simulink model "untitled"  (R2018b)
settings: Solver=VariableStepAuto  StartTime=0.0  StopTime=10.0  RelTol=1e-3
values from neighbouring files (symbols this model uses):
  BOT1_pos = zeros(3,length(t))    [Tetrahedron_Based_Relative_Localization.m]
  bot1_transmitted = zeros(3,length(t))    [Transmission_Channal.m]
  bot2_transmitted = zeros(3,length(t))    [Transmission_Channal.m]
  bot3_transmitted = zeros(3,length(t))    [Transmission_Channal.m]
  bot4_transmitted = zeros(3,length(t))    [Transmission_Channal.m]
undefined symbols (not defined in the file or in its folder): smiData, X, Y, Z
libraries: simulink x15, nesl_utility x6, sm_lib x5
settings Model: Creator=Yogesh  LastModifiedBy=Yogesh

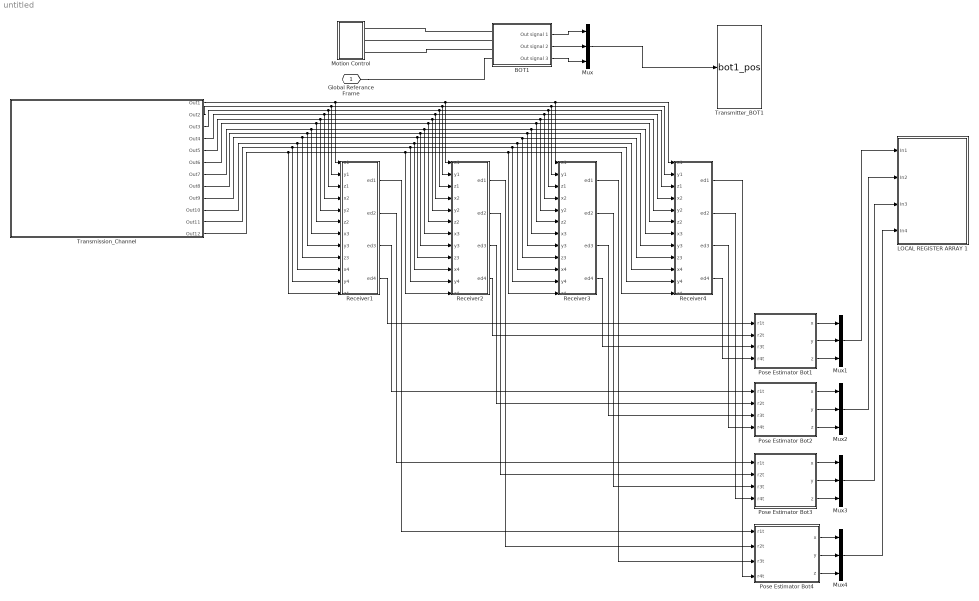
== system untitled ==
  BOT1 : Subsystem
  LOCAL REGISTER ARRAY 1 : Subsystem
  Motion Control : Subsystem
  Mux{,1..4} (5 alike) : Mux  Inputs=3
  Pose Estimator Bot1 : MATLAB Function  TreatAsAtomicUnit=on
  Pose Estimator Bot2 : MATLAB Function  TreatAsAtomicUnit=on
  Pose Estimator Bot3 : MATLAB Function  TreatAsAtomicUnit=on
  Pose Estimator Bot4 : MATLAB Function  TreatAsAtomicUnit=on
  Receiver1 : MATLAB Function  TreatAsAtomicUnit=on
  Receiver2 : MATLAB Function  TreatAsAtomicUnit=on
  Receiver3 : MATLAB Function  TreatAsAtomicUnit=on
  Receiver4 : MATLAB Function  TreatAsAtomicUnit=on
  Transmission_Channel : Subsystem
  Transmitter_BOT1 : ToWorkspace  VariableName=bot1_pos  SampleTime=-1
  Global Referance Frame : PMIOPort  Side=Left
  wires:
  Pose Estimator Bot3/1(x) -> Mux3/1
  Pose Estimator Bot2/1(x) -> Mux2/1
  Pose Estimator Bot3/2(y) -> Mux3/2
  Mux/1 -> Transmitter_BOT1/1
  Mux4/1 -> LOCAL REGISTER ARRAY 1/4(In4)
  Mux2/1 -> LOCAL REGISTER ARRAY 1/2(In2)
  Mux3/1 -> LOCAL REGISTER ARRAY 1/3(In3)
  Mux1/1 -> LOCAL REGISTER ARRAY 1/1(In1)
  Pose Estimator Bot4/3(z) -> Mux4/3
  Pose Estimator Bot2/3(z) -> Mux2/3
  Pose Estimator Bot1/1(x) -> Mux1/1
  Pose Estimator Bot3/3(z) -> Mux3/3
  Pose Estimator Bot4/2(y) -> Mux4/2
  Pose Estimator Bot1/2(y) -> Mux1/2
  Pose Estimator Bot4/1(x) -> Mux4/1
  Pose Estimator Bot2/2(y) -> Mux2/2
  Pose Estimator Bot1/3(z) -> Mux1/3
  BOT1/1(Out signal 1) -> Mux/1
  BOT1/2(Out signal 2) -> Mux/2
  BOT1/3(Out signal 3) -> Mux/3
  Transmission_Channel/6(Out6) -> Receiver1/6(z2), Receiver2/6(z2), Receiver3/6(z2), Receiver4/6(z2)
  Transmission_Channel/4(Out4) -> Receiver1/4(x2), Receiver2/4(x2), Receiver4/4(x2), Receiver3/4(x2)
  Transmission_Channel/2(Out2) -> Receiver1/2(y1), Receiver2/2(y1), Receiver4/2(y1), Receiver3/2(y1)
  Transmission_Channel/11(Out11) -> Receiver1/11(y4), Receiver2/11(y4), Receiver4/11(y4), Receiver3/11(y4)
  Transmission_Channel/3(Out3) -> Receiver1/3(z1), Receiver2/3(z1), Receiver4/3(z1), Receiver3/3(z1)
  Transmission_Channel/1(Out1) -> Receiver1/1(x1), Receiver2/1(x1), Receiver4/1(x1), Receiver3/1(x1)
  Transmission_Channel/9(Out9) -> Receiver1/9(z3), Receiver2/9(z3), Receiver4/9(z3), Receiver3/9(z3)
  Transmission_Channel/5(Out5) -> Receiver1/5(y2), Receiver2/5(y2), Receiver4/5(y2), Receiver3/5(y2)
  Transmission_Channel/12(Out12) -> Receiver1/12(z4), Receiver2/12(z4), Receiver4/12(z4), Receiver3/12(z4)
  Transmission_Channel/10(Out10) -> Receiver1/10(x4), Receiver2/10(x4), Receiver4/10(x4), Receiver3/10(x4)
  Transmission_Channel/8(Out8) -> Receiver1/8(y3), Receiver2/8(y3), Receiver4/8(y3), Receiver3/8(y3)
  Transmission_Channel/7(Out7) -> Receiver1/7(x3), Receiver2/7(x3), Receiver4/7(x3), Receiver3/7(x3)
  Receiver1/1(ed1) -> Pose Estimator Bot4/1(r1t)
  Receiver1/2(ed2) -> Pose Estimator Bot3/1(r1t)
  Receiver1/3(ed3) -> Pose Estimator Bot2/1(r1t)
  Receiver1/4(ed4) -> Pose Estimator Bot1/1(r1t)
  Receiver2/1(ed1) -> Pose Estimator Bot4/2(r2t)
  Receiver2/2(ed2) -> Pose Estimator Bot3/2(r2t)
  Receiver2/3(ed3) -> Pose Estimator Bot2/2(r2t)
  Receiver2/4(ed4) -> Pose Estimator Bot1/2(r2t)
  Receiver3/1(ed1) -> Pose Estimator Bot4/3(r3t)
  Receiver3/2(ed2) -> Pose Estimator Bot3/3(r3t)
  Receiver3/3(ed3) -> Pose Estimator Bot2/3(r3t)
  Receiver3/4(ed4) -> Pose Estimator Bot1/3(r3t)
  Receiver4/1(ed1) -> Pose Estimator Bot4/4(r4t)
  Receiver4/2(ed2) -> Pose Estimator Bot3/4(r4t)
  Receiver4/3(ed3) -> Pose Estimator Bot2/4(r4t)
  Receiver4/4(ed4) -> Pose Estimator Bot1/4(r4t)
  connections:
  BOT1/LConn1 -- Motion Control/RConn1
  BOT1/LConn2 -- Motion Control/RConn2
  BOT1/LConn3 -- Motion Control/RConn3
  Global Referance Frame/RConn1 -- BOT1/LConn4

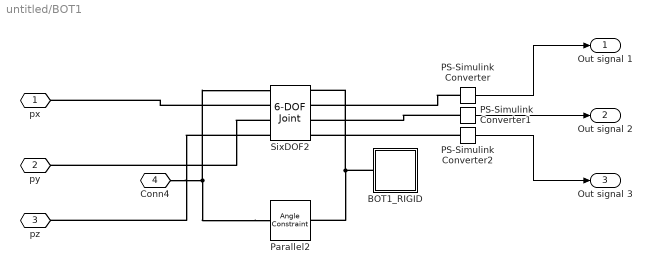
== system untitled/BOT1 ==
  BOT1_RIGID : Subsystem
  PS-Simulink Converter : nesl_utility/PS-Simulink Converter  PhysicalDomain=network_engine_domain  SubClassName=ps_output  LeftPortType=input  RightPortType=output  PseudoPeriodic=off  Frequencies=[]  Unit=m  AffineConversion=off
  PS-Simulink Converter1 : nesl_utility/PS-Simulink Converter  PhysicalDomain=network_engine_domain  SubClassName=ps_output  LeftPortType=input  RightPortType=output  PseudoPeriodic=off  Frequencies=[]  Unit=m  AffineConversion=off
  PS-Simulink Converter2 : nesl_utility/PS-Simulink Converter  PhysicalDomain=network_engine_domain  SubClassName=ps_output  LeftPortType=input  RightPortType=output  PseudoPeriodic=off  Frequencies=[]  Unit=m  AffineConversion=off
  Parallel2 : sm_lib/Constraints/Angle Constraint  ConstraintType=Parallel  Angle=45  AngleUnits=deg  SenseSignedTorqueMagnitude=off  SenseTorque=off  SenseForce=off  WrenchDir=FollowerOnBase  WrenchFrame=BaseFrame
      settings: SourceProductName=Simscape Multibody  SourceProductBaseCode=MS
  SixDOF2 : sm_lib/Joints/6-DOF Joint  SenseConstraintForce=off  SenseConstraintForceX=off  SenseConstraintForceY=off  SenseConstraintForceZ=off  SenseConstraintTorque=off  SenseConstraintTorqueX=off  SenseConstraintTorqueY=off  SenseConstraintTorqueZ=off  SenseTotalForce=off  SenseTotalForceX=off  SenseTotalForceY=off  SenseTotalForceZ=off  SenseTotalTorque=off  SenseTotalTorqueX=off  SenseTotalTorqueY=off  SenseTotalTorqueZ=off  CompositeWrenchDir=FollowerOnBase  CompositeWrenchFrame=BaseFrame  PxEquilibriumPosition=0  PxEquilibriumPositionUnits=m  PxSpringStiffness=0  PxSpringStiffnessUnits=N/m  PxDampingCoefficient=0  PxDampingCoefficientUnits=N/(m/s)  PxTorqueActuationMode=ComputedTorque  PxMotionActuationMode=InputMotion  PxSensePosition=on  PxSenseVelocity=off  PxSenseAcceleration=off  PxSenseTorqueForce=off  PxPositionTargetSpecify=on  PxPositionTargetPriority=Low  PxPositionTargetValue=smiData.SixDofJoint(3).Px.Pos  PxPositionTargetValueUnits=in  PxVelocityTargetSpecify=off  PxVelocityTargetPriority=High  PxVelocityTargetValue=0  PxVelocityTargetValueUnits=m/s  PyEquilibriumPosition=0  PyEquilibriumPositionUnits=m  PySpringStiffness=0  PySpringStiffnessUnits=N/m  PyDampingCoefficient=0  PyDampingCoefficientUnits=N/(m/s)  PyTorqueActuationMode=ComputedTorque  PyMotionActuationMode=InputMotion  PySensePosition=on  PySenseVelocity=off  PySenseAcceleration=off  PySenseTorqueForce=off  PyPositionTargetSpecify=on  PyPositionTargetPriority=Low  PyPositionTargetValue=smiData.SixDofJoint(3).Py.Pos  PyPositionTargetValueUnits=in  PyVelocityTargetSpecify=off  PyVelocityTargetPriority=High  PyVelocityTargetValue=0  PyVelocityTargetValueUnits=m/s  PzEquilibriumPosition=0  PzEquilibriumPositionUnits=m  PzSpringStiffness=0  PzSpringStiffnessUnits=N/m  PzDampingCoefficient=0  PzDampingCoefficientUnits=N/(m/s)  PzTorqueActuationMode=ComputedTorque  PzMotionActuationMode=InputMotion  PzSensePosition=on  PzSenseVelocity=off  PzSenseAcceleration=off  PzSenseTorqueForce=off  PzPositionTargetSpecify=on  PzPositionTargetPriority=Low  PzPositionTargetValue=smiData.SixDofJoint(3).Pz.Pos  PzPositionTargetValueUnits=in  PzVelocityTargetSpecify=off  PzVelocityTargetPriority=High  PzVelocityTargetValue=0  PzVelocityTargetValueUnits=m/s  SphDefPosRotationMethod=None  SphDefPosRotationAngleUnits=deg  SphDefPosRotationStandardAxis=+Z  SphDefPosRotationAngle=0.0  SphDefPosRotationArbitraryAxis=[0 0 1]  SphDefPosFollAlignAxisA=+X  SphDefPosBaseAlignAxisA=+Y  SphDefPosFollAlignAxisB=+Y  SphDefPosBaseAlignAxisB=+Z  SphDefPosRotationSequenceAxes=FollowerAxes  SphDefPosRotationSequence=XYX  SphDefPosRotationSequenceAngles=[0 0 0]  SphDefPosRotationSequenceAnglesUnits=deg  SphDefPosRotationMatrix=[1 0 0; 0 1 0; 0 0 1]  SphEqPosRotationMethod=None  SphEqPosRotationAngleUnits=deg  SphEqPosRotationStandardAxis=+Z  SphEqPosRotationAngle=0.0  SphEqPosRotationArbitraryAxis=[0 0 1]  SphEqPosFollAlignAxisA=+X  SphEqPosBaseAlignAxisA=+Y  SphEqPosFollAlignAxisB=+Y  SphEqPosBaseAlignAxisB=+Z  SphEqPosRotationSequenceAxes=FollowerAxes  SphEqPosRotationSequence=XYX  SphEqPosRotationSequenceAngles=[0 0 0]  SphEqPosRotationSequenceAnglesUnits=deg  SphEqPosRotationMatrix=[1 0 0; 0 1 0; 0 0 1]  SphSpringStiffness=0  SphSpringStiffnessUnits=N*m/rad  SphDampingCoefficient=0  SphDampingCoefficientUnits=N*m/(rad/s)  SphActuateTorqueX=off  SphActuateTorqueY=off  SphActuateTorqueZ=off  SphActuateTorque=off  SphTorqueActuationMode=NoTorque  SphMotionActuationMode=ComputedMotion  SphActuationFrame=BaseFrame  SphSensePosition=off  SphSenseVelocityX=off  SphSenseVelocityY=off  SphSenseVelocityZ=off  SphSenseVelocity=off  SphSenseAccelerationX=off  SphSenseAccelerationY=off  SphSenseAccelerationZ=off  SphSenseAcceleration=off  SphSenseTorqueX=off  SphSenseTorqueY=off  SphSenseTorqueZ=off  SphSenseTorqueForce=off  SphSensingFrame=FollowerFrame  SphPositionTargetRotationMethod=ArbitraryAxis  SphPositionTargetRotationAngleUnits=deg  SphPositionTargetRotationStandardAxis=+Z  SphPositionTargetRotationAngle=smiData.SixDofJoint(3).S.Pos.Angle  SphPositionTargetRotationArbitraryAxis=smiData.SixDofJoint(3).S.Pos.Axis  SphPositionTargetFollAlignAxisA=+X  SphPositionTargetBaseAlignAxisA=+Y  SphPositionTargetFollAlignAxisB=+Y  SphPositionTargetBaseAlignAxisB=+Z  SphPositionTargetRotationSequenceAxes=FollowerAxes  SphPositionTargetRotationSequence=XYX  SphPositionTargetRotationSequenceAngles=[0 0 0]  SphPositionTargetRotationSequenceAnglesUnits=deg  SphPositionTargetRotationMatrix=[1 0 0; 0 1 0; 0 0 1]  SphPositionTargetSpecify=on  SphPositionTargetPriority=Low  SphVelocityTargetValue=[0 0 0]  SphVelocityTargetValueUnits=deg/s  SphVelocityTargetSpecify=off  SphVelocityTargetPriority=High  SphVelocityTargetInFollowerFrame=on
  px : PMIOPort  Side=Left
  py : PMIOPort  Port=2  Side=Left
  pz : PMIOPort  Port=3  Side=Left
  Conn4 : PMIOPort  Port=4  Side=Left
  Out signal 1 : Outport
  Out signal 2 : Outport  Port=2
  Out signal 3 : Outport  Port=3
  wires:
  PS-Simulink Converter/1 -> Out signal 1/1
  PS-Simulink Converter1/1 -> Out signal 2/1
  PS-Simulink Converter2/1 -> Out signal 3/1
  connections:
  SixDOF2/RConn1 -- BOT1_RIGID/LConn1 -- Parallel2/RConn1
  SixDOF2/LConn2 -- px/RConn1
  PS-Simulink Converter1/LConn1 -- SixDOF2/RConn3
  Parallel2/LConn1 -- Conn4/RConn1 -- SixDOF2/LConn1
  PS-Simulink Converter/LConn1 -- SixDOF2/RConn2
  PS-Simulink Converter2/LConn1 -- SixDOF2/RConn4
  SixDOF2/LConn3 -- py/RConn1
  SixDOF2/LConn4 -- pz/RConn1

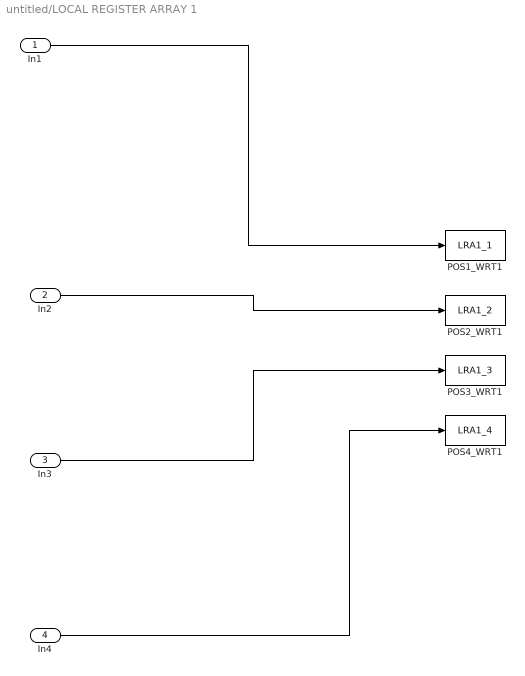
== system untitled/LOCAL REGISTER ARRAY 1 ==
  In1 : Inport
  In2 : Inport  Port=2
  In3 : Inport  Port=3
  In4 : Inport  Port=4
  POS1_WRT1 : ToWorkspace  VariableName=LRA1_1  SampleTime=-1
  POS2_WRT1 : ToWorkspace  VariableName=LRA1_2  SampleTime=-1
  POS3_WRT1 : ToWorkspace  VariableName=LRA1_3  SampleTime=-1
  POS4_WRT1 : ToWorkspace  VariableName=LRA1_4  SampleTime=-1
  wires:
  In2/1 -> POS2_WRT1/1
  In3/1 -> POS3_WRT1/1
  In1/1 -> POS1_WRT1/1
  In4/1 -> POS4_WRT1/1

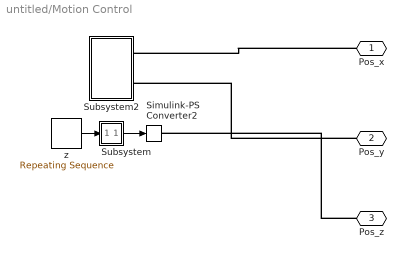
== system untitled/Motion Control ==
  Simulink-PS Converter2 : nesl_utility/Simulink-PS Converter  PhysicalDomain=network_engine_domain  SubClassName=ps_input  LeftPortType=input  RightPortType=output  PseudoPeriodic=off  Frequencies=[]  NoiseDistribution=none  NoiseParameters=[]  Unit=m  AffineConversion=off  FilteringAndDerivatives=filter  SimscapeFilterOrder=2  InputFilterTimeConstant=0.001  UdotUserProvided=0
  Subsystem : Subsystem
  Subsystem2 : Subsystem
  z : simulink/Sources/Repeating Sequence  rep_seq_t=t  rep_seq_y=BOT1_pos(3,:)
  Pos_x : PMIOPort  Side=Right
  Pos_y : PMIOPort  Port=2  Side=Right
  Pos_z : PMIOPort  Port=3  Side=Right
  wires:
  Subsystem/1(2) -> Simulink-PS Converter2/1
  z/1 -> Subsystem/1(1)
  connections:
  Pos_z/RConn1 -- Simulink-PS Converter2/RConn1
  Pos_y/RConn1 -- Subsystem2/RConn2
  Pos_x/RConn1 -- Subsystem2/RConn1

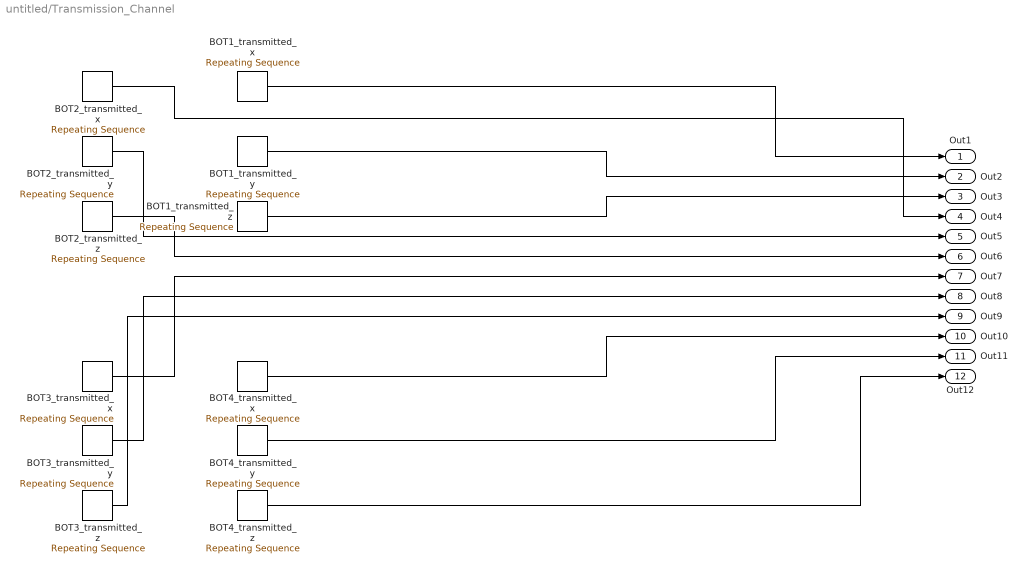
== system untitled/Transmission_Channel ==
  BOT1_transmitted_x : simulink/Sources/Repeating Sequence  rep_seq_t=t  rep_seq_y=bot1_transmitted(1,:)
  BOT1_transmitted_y : simulink/Sources/Repeating Sequence  rep_seq_t=t  rep_seq_y=bot1_transmitted(2,:)
  BOT1_transmitted_z : simulink/Sources/Repeating Sequence  rep_seq_t=t  rep_seq_y=bot1_transmitted(3,:)
  BOT2_transmitted_x : simulink/Sources/Repeating Sequence  rep_seq_t=t  rep_seq_y=bot2_transmitted(1,:)
  BOT2_transmitted_y : simulink/Sources/Repeating Sequence  rep_seq_t=t  rep_seq_y=bot2_transmitted(2,:)
  BOT2_transmitted_z : simulink/Sources/Repeating Sequence  rep_seq_t=t  rep_seq_y=bot2_transmitted(3,:)
  BOT3_transmitted_x : simulink/Sources/Repeating Sequence  rep_seq_t=t  rep_seq_y=bot3_transmitted(1,:)
  BOT3_transmitted_y : simulink/Sources/Repeating Sequence  rep_seq_t=t  rep_seq_y=bot3_transmitted(2,:)
  BOT3_transmitted_z : simulink/Sources/Repeating Sequence  rep_seq_t=t  rep_seq_y=bot3_transmitted(3,:)
  BOT4_transmitted_x : simulink/Sources/Repeating Sequence  rep_seq_t=t  rep_seq_y=bot4_transmitted(1,:)
  BOT4_transmitted_y : simulink/Sources/Repeating Sequence  rep_seq_t=t  rep_seq_y=bot4_transmitted(2,:)
  BOT4_transmitted_z : simulink/Sources/Repeating Sequence  rep_seq_t=t  rep_seq_y=bot4_transmitted(3,:)
  Out1 : Outport
  Out2 : Outport  Port=2
  Out3 : Outport  Port=3
  Out4 : Outport  Port=4
  Out5 : Outport  Port=5
  Out6 : Outport  Port=6
  Out7 : Outport  Port=7
  Out8 : Outport  Port=8
  Out9 : Outport  Port=9
  Out10 : Outport  Port=10
  Out11 : Outport  Port=11
  Out12 : Outport  Port=12
  wires:
  BOT1_transmitted_x/1 -> Out1/1
  BOT4_transmitted_z/1 -> Out12/1
  BOT1_transmitted_z/1 -> Out3/1
  BOT3_transmitted_x/1 -> Out7/1
  BOT3_transmitted_z/1 -> Out9/1
  BOT2_transmitted_z/1 -> Out6/1
  BOT2_transmitted_y/1 -> Out5/1
  BOT3_transmitted_y/1 -> Out8/1
  BOT1_transmitted_y/1 -> Out2/1
  BOT2_transmitted_x/1 -> Out4/1
  BOT4_transmitted_x/1 -> Out10/1
  BOT4_transmitted_y/1 -> Out11/1

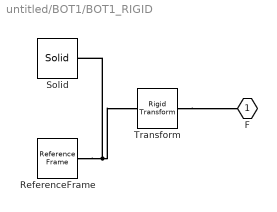
== system untitled/BOT1/BOT1_RIGID ==
  ReferenceFrame : sm_lib/Frames and Transforms/Reference Frame
  Solid : sm_lib/Body Elements/Solid  InertiaType=Custom  Mass=smiData.Solid(3).mass  MassUnits=kg  CenterOfMass=smiData.Solid(3).CoM  CenterOfMassUnits=mm  MomentsOfInertia=smiData.Solid(3).MoI  MomentsOfInertiaUnits=kg*mm^2  ProductsOfInertia=smiData.Solid(3).PoI  ProductsOfInertiaUnits=kg*mm^2  BasedOnType=Density  Density=1000  DensityUnits=kg/m^3  DoExposeReferenceFrame=on  SerializedFrames=<Frames/>  GraphicType=FromGeometry  MarkerShape=Sphere  MarkerSize=10  GraphicVisPropType=AdvancedVisualProperties  GraphicDiffuseColor=[1.0 0.2 0.2]  GraphicSpecularColor=[0.5 0.5 0.5 1.0]  GraphicAmbientColor=[0.15 0.15 0.15 1.0]  GraphicEmissiveColor=[0.0 0.0 0.0 1.0]  GraphicShininess=75  GraphicOpacity=smiData.Solid(3).opacity  GeometryShape=FromFile  RectangleSize=[1 1]  RectangleSizeUnits=m  BrickDimensions=[1 1 1]  BrickDimensionUnits=m  CylinderRadius=1  CylinderRadiusUnits=m  CylinderLength=1  CylinderLengthUnits=m  SphereRadius=1  SphereRadiusUnits=m  EllipsoidRadii=[1 1 1]  EllipsoidRadiiUnits=m  ExtrusionCrossSection=[1 1; -1 1; -1 -1; 1 -1]  ExtrusionCrossSectionUnits=m  ExtrusionLength=1  ExtrusionLengthUnits=m  PolygonNumSides=3  PolygonOuterRadius=1  PolygonOuterRadiusUnits=m  ExtGeomFileType=STEP  ExtGeomFileName=BOT3_Default_sldprt.STEP  ExtGeomFileUnits=m  RevolutionCrossSection=[1 1; 1 -1; 2 -1; 2 1]  RevolutionCrossSectionUnits=m  RevolutionExtent=Full  RevolutionAngle=180  RevolutionAngleUnits=deg
  Transform : sm_lib/Frames and Transforms/Rigid Transform  TranslationMethod=Cartesian  TranslationStandardOffset=0  TranslationLengthUnit=m  TranslationStandardAxis=+Z  TranslationCartesianOffset=smiData.RigidTransform(6).translation  TranslationROffset=0  TranslationROffsetUnits=m  TranslationZOffset=0  TranslationZOffsetUnits=m  TranslationThetaOffset=0  TranslationThetaOffsetUnits=deg  RotationMethod=ArbitraryAxis  RotationAngleUnits=rad  RotationStandardAxis=+Z  RotationAngle=smiData.RigidTransform(6).angle  RotationArbitraryAxis=smiData.RigidTransform(6).axis  FollAlignAxisA=+X  BaseAlignAxisA=+Y  FollAlignAxisB=+Y  BaseAlignAxisB=+Z  RotationSequenceAxes=FollowerAxes  RotationSequence=XYX  RotationSequenceAngles=[0 0 0]  RotationSequenceAnglesUnits=deg  RotationMatrix=[1 0 0; 0 1 0; 0 0 1]
  F : PMIOPort  Side=Left
  connections:
  Solid/RConn1 -- ReferenceFrame/RConn1 -- Transform/LConn1
  Transform/RConn1 -- F/RConn1

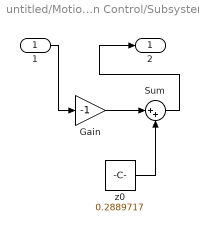
== system untitled/Motion Control/Subsystem ==
  1 : Inport
  Gain : Gain  Gain=-1
  Sum : Sum  Inputs=|++
  z0 : Constant  Value=0.2889717
  2 : Outport
  wires:
  z0/1 -> Sum/2
  Gain/1 -> Sum/1
  Sum/1 -> 2/1
  1/1 -> Gain/1

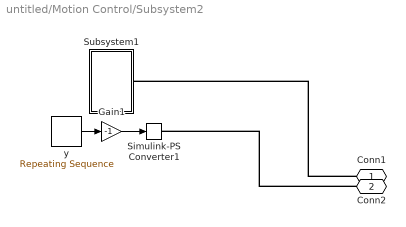
== system untitled/Motion Control/Subsystem2 ==
  Gain1 : Gain  Gain=-1
  Simulink-PS Converter1 : nesl_utility/Simulink-PS Converter  PhysicalDomain=network_engine_domain  SubClassName=ps_input  LeftPortType=input  RightPortType=output  PseudoPeriodic=off  Frequencies=[]  NoiseDistribution=none  NoiseParameters=[]  Unit=m  AffineConversion=off  FilteringAndDerivatives=filter  SimscapeFilterOrder=2  InputFilterTimeConstant=0.001  UdotUserProvided=0
  Subsystem1 : Subsystem
  y : simulink/Sources/Repeating Sequence  rep_seq_t=t  rep_seq_y=BOT1_pos(2,:)
  Conn1 : PMIOPort  Side=Right
  Conn2 : PMIOPort  Port=2  Side=Right
  wires:
  y/1 -> Gain1/1
  Gain1/1 -> Simulink-PS Converter1/1
  connections:
  Conn2/RConn1 -- Simulink-PS Converter1/RConn1
  Conn1/RConn1 -- Subsystem1/RConn1

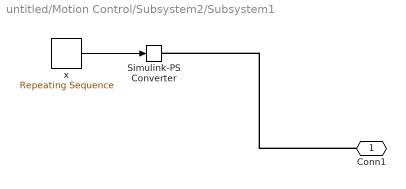
== system untitled/Motion Control/Subsystem2/Subsystem1 ==
  Simulink-PS Converter : nesl_utility/Simulink-PS Converter  PhysicalDomain=network_engine_domain  SubClassName=ps_input  LeftPortType=input  RightPortType=output  PseudoPeriodic=off  Frequencies=[]  NoiseDistribution=none  NoiseParameters=[]  Unit=m  AffineConversion=off  FilteringAndDerivatives=filter  SimscapeFilterOrder=2  InputFilterTimeConstant=0.001  UdotUserProvided=0
  x : simulink/Sources/Repeating Sequence  rep_seq_t=t  rep_seq_y=BOT1_pos(1,:)
  Conn1 : PMIOPort  Side=Right
  wires:
  x/1 -> Simulink-PS Converter/1
  connections:
  Conn1/RConn1 -- Simulink-PS Converter/RConn1

== matlab function untitled/Receiver2 ==
  data: x1 input; ed1 output; y1 input; z1 input; x2 input; y2 input; z2 input; x3 input; y3 input; z3 input; x4 input; y4 input; z4 input; ed2 output; ed3 output; ed4 output
function [ed1,ed2,ed3,ed4] = fcn(x1,y1,z1,x2,y2,z2,x3,y3,z3,x4,y4,z4)
ed1 = ((x1-x1)^2+(y1-0.57735-y1)^2+(z1+0.204124-z1)^2)^0.5;
ed2 = ((x2-x1)^2+(y2-0.57735-y1)^2+(z2+0.204124-z1)^2)^0.5;
ed3 = ((x3-x1)^2+(y3-0.57735-y1)^2+(z3+0.204124-z1)^2)^0.5;
ed4 = ((x4-x1)^2+(y4-0.57735-y1)^2+(z4+0.204124-z1)^2)^0.5;

== matlab function untitled/Receiver3 ==
  data: x1 input; ed1 output; y1 input; z1 input; x2 input; y2 input; z2 input; x3 input; y3 input; z3 input; x4 input; y4 input; z4 input; ed2 output; ed3 output; ed4 output
function [ed1,ed2,ed3,ed4] = fcn(x1,y1,z1,x2,y2,z2,x3,y3,z3,x4,y4,z4)
ed1 = ((x1-x1)^2+(y1-0.57735-y1)^2+(z1+0.204124-z1)^2)^0.5;
ed2 = ((x2-x1)^2+(y2-0.57735-y1)^2+(z2+0.204124-z1)^2)^0.5;
ed3 = ((x3-x1)^2+(y3-0.57735-y1)^2+(z3+0.204124-z1)^2)^0.5;
ed4 = ((x4-x1)^2+(y4-0.57735-y1)^2+(z4+0.204124-z1)^2)^0.5;

== matlab function untitled/Receiver4 ==
  data: x1 input; ed1 output; y1 input; z1 input; x2 input; y2 input; z2 input; x3 input; y3 input; z3 input; x4 input; y4 input; z4 input; ed2 output; ed3 output; ed4 output
function [ed1,ed2,ed3,ed4] = fcn(x1,y1,z1,x2,y2,z2,x3,y3,z3,x4,y4,z4)
ed1 = ((x1-x1)^2+(y1-0.57735-y1)^2+(z1+0.204124-z1)^2)^0.5;
ed2 = ((x2-x1)^2+(y2-0.57735-y1)^2+(z2+0.204124-z1)^2)^0.5;
ed3 = ((x3-x1)^2+(y3-0.57735-y1)^2+(z3+0.204124-z1)^2)^0.5;
ed4 = ((x4-x1)^2+(y4-0.57735-y1)^2+(z4+0.204124-z1)^2)^0.5;

== matlab function untitled/Pose Estimator Bot1 ==
  data: x output; r1t input; y output; r2t input; r3t input; r4t input; z output
function [x,y,z] = fcn(r1t,r2t,r3t,r4t)
M = [0 -3.8462 0;4.4412 2.2206 0;-1.5702 -3.3140 -4.7104];
R = [r2t^2-r1t^2;r3t^2-r2t^2;r4t^2-r3t^2];
P = M*R;
x = P(1);
y = P(2);
z = P(3);

== matlab function untitled/Pose Estimator Bot2 ==
  data: x output; r1t input; y output; r2t input; r3t input; r4t input; z output
function [x,y,z] = fcn(r1t,r2t,r3t,r4t)
M = [0 -3.8462 0;4.4412 2.2206 0;-1.5702 -3.3140 -4.7104];
R = [r2t^2-r1t^2;r3t^2-r2t^2;r4t^2-r3t^2];
P = M*R;
x = P(1);
y = P(2);
z = P(3);

== matlab function untitled/Pose Estimator Bot3 ==
  data: x output; r1t input; y output; r2t input; r3t input; r4t input; z output
function [x,y,z] = fcn(r1t,r2t,r3t,r4t)
M = [0 -3.8462 0;4.4412 2.2206 0;-1.5702 -3.3140 -4.7104];
R = [r2t^2-r1t^2;r3t^2-r2t^2;r4t^2-r3t^2];
P = M*R;
x = P(1);
y = P(2);
z = P(3);

== matlab function untitled/Pose Estimator Bot4 ==
  data: x output; r1t input; y output; r2t input; r3t input; r4t input; z output
function [x,y,z] = fcn(r1t,r2t,r3t,r4t)
M = [0 -3.8462 0;4.4412 2.2206 0;-1.5702 -3.3140 -4.7104];
R = [r2t^2-r1t^2;r3t^2-r2t^2;r4t^2-r3t^2];
P = M*R;
x = P(1);
y = P(2);
z = P(3);

== matlab function untitled/Receiver1 ==
  data: x1 input; ed1 output; y1 input; z1 input; x2 input; y2 input; z2 input; x3 input; y3 input; z3 input; x4 input; y4 input; z4 input; ed2 output; ed3 output; ed4 output
function [ed1,ed2,ed3,ed4] = fcn(x1,y1,z1,x2,y2,z2,x3,y3,z3,x4,y4,z4)
ed1 = ((x1-x1)^2+(y1-0.57735-y1)^2+(z1+0.204124-z1)^2)^0.5;
ed2 = ((x2-x1)^2+(y2-0.57735-y1)^2+(z2+0.204124-z1)^2)^0.5;
ed3 = ((x3-x1)^2+(y3-0.57735-y1)^2+(z3+0.204124-z1)^2)^0.5;
ed4 = ((x4-x1)^2+(y4-0.57735-y1)^2+(z4+0.204124-z1)^2)^0.5;
